simulink model "Intergration"  (R2018b)
settings: Solver=FixedStepDiscrete  StartTime=0.0  StopTime=inf  FixedStep=0.005  RelTol=1e-3
PostLoadFcn:
  | if any(exist('dsrtsu_mdlpostloadfcn', 'file') ~= 0), dsrtsu_mdlpostloadfcn('Execute', bdroot); end
values from neighbouring files (symbols this model uses):
  P_x165_On = 1.0    [CAN_Tx.sldd]
  P_x242_On = 1.0    [CAN_Tx.sldd]
  P_x246_On = 1.0    [CAN_Tx.sldd]
libraries: rtican x112, simulink x59
(part 13 of 31)

== system Intergration/Radar410_RX/x61_31 ==
  Bus Creator1 : BusCreator  Inputs=20
  FRS_Obj_17_Part1of2 : rtican/RTICAN Receive (RX)   Reserved1=[]  Reserved2=[]  Reserved3=[]  Reserved4=[]  SfcnMessage=[]  Msg_Struct=[]  BoardTypeNo=[]  BoardNo=[]  ChannelNo=[]  Parameters=[]  DialogFcn=[]  UnitName=[]  Revision=[]  UnitValues=[]  DSProperties=struct('RTI',struct('Version',uint32(5),'BlockType',struct('isSLSource',uint8(1),'isSLSink',uint8(1),'isHWSource',uint8(0),'isHWSink',uint8(0),'isSetup',uint8(0),'isInline',uint8(1),'isNonInline',uint8(0),'isInterrupt',uint8(0),'isChannelwise',uint8(0)),'IOBoardType','RTICAN','UnitType','MESSAGE','Identifier','RX','DialogType','MSVC','BlockSet','RTICAN','SlaveProcessor','CAN'))  RTIBlockInterface=struct('OutputPortsWidth',int32([1 1 1 1 1 1 1 1 1 1 1 1 1 1 1]),'OutputPortsActive',ones(1,15),'OutputPortsName',{{'FRS_P1_17_Msg_CheckSum','FRS_P1_17_Msg_AliveCounter','FRS_P1_17_Obj_ExstProb','FRS_P1_17_Obj_XVelRel_Stdev','FRS_P1_17_Obj_XAccRel','FRS_P1_17_Obj_ObstacleProb','FRS_P1_17_Obj_MotionPattern','FRS_P1_17_Obj_YPos_Stdev','FRS_P1_17_Obj_ValidFlag','FRS_P1_17_Obj_XPos_Stdev','FRS_P1_17_Obj_UpdateFlag','FRS_P1_17_Obj_ID',['RX status'],['RX time'],['RX delta time']}},'OutputPortsDataType',{{'SS_DOUBLE','SS_DOUBLE','SS_DOUBLE','SS_DOUBLE','SS_DOUBLE','SS_DOUBLE','SS_DOUBLE','SS_DOUBLE','SS_DOUBLE','SS_DOUBLE','SS_DOUBLE','SS_DOUBLE','SS_DOUBLE','SS_DOUBLE','SS_DOUBLE'}},'OutputPortsLabel',{{'FRS_P1_17_Msg_CheckSum','FRS_P1_17_Msg_AliveCounter','FRS_P1_17_Obj_ExstProb','FRS_P1_17_Obj_XVelRel_Stdev','FRS_P1_17_Obj_XAccRel','FRS_P1_17_Obj_ObstacleProb','FRS_P1_17_Obj_MotionPattern','FRS_P1_17_Obj_YPos_Stdev','FRS_P1_17_Obj_ValidFlag','FRS_P1_17_Obj_XPos_Stdev','FRS_P1_17_Obj_UpdateFlag','FRS_P1_17_Obj_ID','','',''}},'OutputPortsLabelMode','ON','InputPortsWidth',int32(0),'InputPortsActive',0,'DialogFcn','rtican_message_interface_gui','BlockDisplay',{{'','center'}},'IconTransparency','on','ParameterTunableNames',{{}},'InitLevel',3,'BlockName',struct('Token',{{'FRS_Obj_17_Part1of2'}}),'SampleTime',{{-1}},'TriggerPort',{{'none'}},'EnablePort',{{'none'}})  RTIBlockParameters=struct('BoardTypeNo',{{1,'OFF',[]}},'BoardNo',{{2,'ON',[1 16]}},'ChannelNo',{{2,'ON',[1 2]}},'Parameters',{{struct('DataFileSupport',struct('DataFileSelectedMaster',1,'DataFileSelectedLocal',1,'DataFileName','d:\00_work\00_zop\00_zop_demo_sim\asr410od_privatecan\privatecan\ars410od_privatecan.dbc|','DataFileDate',{{{['04-12月-2019 16:27:24']}}},'SelectedFile','asr410od_privatecan\privatecan\ars410od_privatecan.dbc'),'Options',struct('StatusSelected',1,'TimeSelected',1,'DeltaTimeSelected',1,'BytePortSelected',0,'MessageLengthSelected',0,'TriggerPort',struct('Selected',0,'TriggerType',0),'UserCoding',struct('Selected',0,'InterfaceFile','UserDecodingFile','FcnName','UserDecodeFcn','InportSelected',0,'InportWidth',1,'OutportSelected',0,'OutportWidth',1),'EnablePortSelected',0,'SignalOnPortnameSelected',1,'UseRXService',0),'Message',struct('MsgOnBlocknameSelected',1,'MsgName','FRS_Obj_17_Part1of2','MsgIdFormat',0,'MsgId',97,'MsgLength',8,'NumSignals',12,'SampleTime',-1,'Signal',struct('SgnName',{'FRS_P1_17_Msg_CheckSum','FRS_P1_17_Msg_AliveCounter','FRS_P1_17_Obj_ExstProb','FRS_P1_17_Obj_XVelRel_Stdev','FRS_P1_17_Obj_XAccRel','FRS_P1_17_Obj_ObstacleProb','FRS_P1_17_Obj_MotionPattern','FRS_P1_17_Obj_YPos_Stdev','FRS_P1_17_Obj_ValidFlag','FRS_P1_17_Obj_XPos_Stdev','FRS_P1_17_Obj_UpdateFlag','FRS_P1_17_Obj_ID'},'SgnStartBit',{0,8,12,18,25,32,37,40,47,48,55,56},'SgnLength',{8,4,6,7,7,5,3,7,1,7,1,8},'SgnType',{0,0,0,0,0,0,0,0,0,0,0,0},'ModeValue',{-1,-1,-1,-1,-1,-1,-1,-1,-1,-1,-1,-1},'DataType',{0,0,0,0,0,0,0,0,0,0,0,0},'ByteLayout',{2,2,2,2,2,2,2,2,2,2,2,2},'Factor',{1,1,1.5873,0.05,0.15,3.2258,1,0.1,1,0.1,1,1},'Offset',{0,0,0,0,-9.6,0,0,0,0,0,0,0},'SgnComment',{{['Check sum shall be generated out of each message content. check sum generation logic is TBC.']},{['Alive counter shall be incremented every radar sensor measurement cycle.']},{['Estimated existence probability of the object.']},{['Estimated 3-sigma standard deviation value of the relative longitudinal velocity of the object.']},{['Relative longitudinal acceleration of the object']},{['Estimated probability of the object being an obstacle.']},{['Motion type of object.' char(10) '0x00: Unknown' char(10) '0x01: Stationary' char(10) '0x02: Stopped' char(10) '0x03: Moving' char(10) '0x04: Crossing' char(10) '0x05-07: reserved']},{['Estimated 3-sigma standard deviation value of lateral position of the object.']},{['Validity indication flag. when this value shows invalid, all the signals in the corresponding CAN messages except FRS_Msg_AliveCounter and FRS_Msg_CheckSum shall take default values.' char(10) '0x0: Object invalid' char(10) '0x1: Object valid']},{['Estimated 3-sigma standard deviation value of longitudinal position of the object.']},{['Flag to indicate newly created object in CAN bus.' char(10) 'Object history flag' char(10) '0x0: new object in the cycle;' char(10) '0x1: object existed in previous cycle']},{['ID is defined as a unique identification number over the lifetime of the object.' char(10) '0xFF: Invalid' char(10) '0x00 - 0xFE: Valid']}},'SgnUnit',{'n/a','n/a','%','m/s','m/s2','%','n/a','m','n/a','m','n/a','n/a'},'Min',{0,0,0,0,-9.6,0,0,0,0,0,0,0},'Max',{255,15,99.9999,6.35,9.45,99.9998,7,12.7,1,12.7,1,255},'SLDataType',{'SS_DOUBLE','SS_DOUBLE','SS_DOUBLE','SS_DOUBLE','SS_DOUBLE','SS_DOUBLE','SS_DOUBLE','SS_DOUBLE','SS_DOUBLE','SS_DOUBLE','SS_DOUBLE','SS_DOUBLE'}),'MsgIdNumFormat',0,'MsgComment',{{''}}),'Version',1.2,'general',struct('isFromLib',0)),'OFF',[]}},'GroupId',{{struct('Group',{{'RTICAN'}},'No',2,'Behavior',{{'NAMECHANGE'}},'BlockType',{{'SINK'}},'NameChangeFlag',0),'OFF',[]}},'SFcnRTICANMessage',{{struct('MsgType','RX','SFcnPortType','Scalar','MsgName','FRS_Obj_17_Part1of2','MsgIdFormat','STD','MsgId',97,'MsgLength',8,'NumSignals',12,'SampleTime',-1,'Signal',struct('SgnName',{'FRS_P1_17_Msg_CheckSum','FRS_P1_17_Msg_AliveCounter','FRS_P1_17_Obj_ExstProb','FRS_P1_17_Obj_XVelRel_Stdev','FRS_P1_17_Obj_XAccRel','FRS_P1_17_Obj_ObstacleProb','FRS_P1_17_Obj_MotionPattern','FRS_P1_17_Obj_YPos_Stdev','FRS_P1_17_Obj_ValidFlag','FRS_P1_17_Obj_XPos_Stdev','FRS_P1_17_Obj_UpdateFlag','FRS_P1_17_Obj_ID'},'SgnStartBit',{0,8,12,18,25,32,37,40,47,48,55,56},'SgnLength',{8,4,6,7,7,5,3,7,1,7,1,8},'SgnType',{'standard','standard','standard','standard','standard','standard','standard','standard','standard','standard','standard','standard'},'ModeValue',{-1,-1,-1,-1,-1,-1,-1,-1,-1,-1,-1,-1},'DataType',{['unsigned int'],['unsigned int'],['unsigned int'],['unsigned int'],['unsigned int'],['unsigned int'],['unsigned int'],['unsigned int'],['unsigned int'],['unsigned int'],['unsigned int'],['unsigned int']},'ByteLayout',{['motorola back.'],['motorola back.'],['motorola back.'],['motorola back.'],['motorola back.'],['motorola back.'],['motorola back.'],['motorola back.'],['motorola back.'],['motorola back.'],['motorola back.'],['motorola back.']},'Factor',{1,1,1.5873,0.05,0.15,3.2258,1,0.1,1,0.1,1,1},'Offset',{0,0,0,0,-9.6,0,0,0,0,0,0,0},'SLDataType',{'SS_DOUBLE','SS_DOUBLE','SS_DOUBLE','SS_DOUBLE','SS_DOUBLE','SS_DOUBLE','SS_DOUBLE','SS_DOUBLE','SS_DOUBLE','SS_DOUBLE','SS_DOUBLE','SS_DOUBLE'}),'StatusSelected','yes','TimeSelected','yes','DeltaTimeSelected','yes','BytePortSelected','no','MessageLengthSelected','no','TriggerPort',struct('Selected','no','TriggerType',0),'UserCoding',struct('Selected','no','InterfaceFile','UserDecodingFile','FcnName','UserDecodeFcn','InportSelected','no','InportWidth',1,'OutportSelected','no','OutportWidth',1),'EnablePortSelected','no','UseRXService','no','BoardType','DS1','BoardNo',2,'ControllerNo',1),'OFF',[]}},'TLCFileName',{{'rtican_rx_message','OFF',[]}})  RTISFcnParameters=struct('SFcnRTICANMessage','struct','TLCFileName','char')  RTIBlockParaDefault=struct('BoardTypeNo',4302,'BoardNo',1,'ChannelNo',1,'Parameters',struct('DataFileSupport',struct('DataFileSelectedMaster',0,'DataFileSelectedLocal',0,'DataFileName','','DataFileDate','','SelectedFile',['<no file selected>']),'Options',struct('StatusSelected',1,'TimeSelected',1,'DeltaTimeSelected',1,'BytePortSelected',0,'MessageLengthSelected',0,'TriggerPort',struct('Selected',0,'TriggerType','rising'),'UserCoding',struct('Selected',0,'InterfaceFile','UserDecodingFile','FcnName','UserDecodeFcn','InportSelected',0,'InportWidth',1,'OutportSelected',0,'OutportWidth',1),'EnablePortSelected',0,'SignalOnPortnameSelected',1,'UseRXService',0),'Message',struct('MsgOnBlocknameSelected',0,'MsgName',['RX Message'],'MsgIdFormat',0,'MsgId',100,'MsgLength',8,'NumSignals',1,'SampleTime',-1,'Signal',struct('SgnName',['RX signal'],'SgnStartBit',0,'SgnLength',8,'SgnType',0,'ModeValue',-1,'DataType',0,'SLDataType','SS_DOUBLE','ByteLayout',0,'Factor',1,'Offset',0,'Min',0,'Max',255,'SgnComment',{{}},'SgnUnit',''),'MsgIdNumFormat',0,'MsgComment',{{''}}),'Version',1.2,'general',struct('isFromLib',1)),'GroupId',struct('Group',{{'RTICAN'}},'No',1,'Behavior',{{'NAMECHANGE'}},'BlockType',{{'SINK'}},'NameChangeFlag',0),'SFcnRTICANMessage',struct('MsgType','RX','MsgName',['RX Message'],'MsgIdFormat','STD','MsgId',100,'MsgLength',8,'NumSignals',1,'SampleTime',-1,'Signal',struct('SgnName',['RX signal'],'SgnStartBit',0,'SgnLength',8,'SgnType','standard','ModeValue',-1,'DataType',['unsigned int'],'ByteLayout',['little endian'],'SLDataType','SS_DOUBLE','Factor',1,'Offset',0),'StatusSelected','yes','TimeSelected','yes','DeltaTimeSelected','yes','BytePortSelected','no','MessageLengthSelected','no','EnablePortSelected','no','UserCoding',struct('Selected','no','InterfaceFile','UserDecodingFile','FcnName','UserDecodeFcn','InportSelected','no','InportWidth',1,'OutportSelected','no','OutportWidth',1),'TriggerPort',struct('Selected','no','TriggerType','rising'),'UseRXService','no','BoardType','DS4302','BoardNo',1,'ControllerNo',1,'SFcnPortType','Scalar'),'TLCFileName','rtican_rx_message')
      settings: AttributesFormatString=Group Id: RTICAN2\n  SourceProductName=dSPACE RTI CAN Blockset
  FRS_Obj_17_Part2of2 : rtican/RTICAN Receive (RX)   Reserved1=[]  Reserved2=[]  Reserved3=[]  Reserved4=[]  SfcnMessage=[]  Msg_Struct=[]  BoardTypeNo=[]  BoardNo=[]  ChannelNo=[]  Parameters=[]  DialogFcn=[]  UnitName=[]  Revision=[]  UnitValues=[]  DSProperties=struct('RTI',struct('Version',uint32(5),'BlockType',struct('isSLSource',uint8(1),'isSLSink',uint8(1),'isHWSource',uint8(0),'isHWSink',uint8(0),'isSetup',uint8(0),'isInline',uint8(1),'isNonInline',uint8(0),'isInterrupt',uint8(0),'isChannelwise',uint8(0)),'IOBoardType','RTICAN','UnitType','MESSAGE','Identifier','RX','DialogType','MSVC','BlockSet','RTICAN','SlaveProcessor','CAN'))  RTIBlockInterface=struct('OutputPortsWidth',int32([1 1 1 1 1 1 1 1 1 1 1]),'OutputPortsActive',ones(1,11),'OutputPortsName',{{'FRS_P2_17_Msg_CheckSum','FRS_P2_17_Msg_AliveCounter','FRS_P2_17_Obj_MeasFlag','FRS_P2_17_Obj_YVelRel','FRS_P2_17_Obj_Type','FRS_P2_17_Obj_XPos','FRS_P2_17_Obj_YPos','FRS_P2_17_Obj_XVelRel',['RX status'],['RX time'],['RX delta time']}},'OutputPortsDataType',{{'SS_DOUBLE','SS_DOUBLE','SS_DOUBLE','SS_DOUBLE','SS_DOUBLE','SS_DOUBLE','SS_DOUBLE','SS_DOUBLE','SS_DOUBLE','SS_DOUBLE','SS_DOUBLE'}},'OutputPortsLabel',{{'FRS_P2_17_Msg_CheckSum','FRS_P2_17_Msg_AliveCounter','FRS_P2_17_Obj_MeasFlag','FRS_P2_17_Obj_YVelRel','FRS_P2_17_Obj_Type','FRS_P2_17_Obj_XPos','FRS_P2_17_Obj_YPos','FRS_P2_17_Obj_XVelRel','','',''}},'OutputPortsLabelMode','ON','InputPortsWidth',int32(0),'InputPortsActive',0,'DialogFcn','rtican_message_interface_gui','BlockDisplay',{{'','center'}},'IconTransparency','on','ParameterTunableNames',{{}},'InitLevel',3,'BlockName',struct('Token',{{'FRS_Obj_17_Part2of2'}}),'SampleTime',{{-1}},'TriggerPort',{{'none'}},'EnablePort',{{'none'}})  RTIBlockParameters=struct('BoardTypeNo',{{1,'OFF',[]}},'BoardNo',{{2,'ON',[1 16]}},'ChannelNo',{{2,'ON',[1 2]}},'Parameters',{{struct('DataFileSupport',struct('DataFileSelectedMaster',1,'DataFileSelectedLocal',1,'DataFileName','d:\00_work\00_zop\00_zop_demo_sim\asr410od_privatecan\privatecan\ars410od_privatecan.dbc|','DataFileDate',{{{['04-12月-2019 16:27:24']}}},'SelectedFile','asr410od_privatecan\privatecan\ars410od_privatecan.dbc'),'Options',struct('StatusSelected',1,'TimeSelected',1,'DeltaTimeSelected',1,'BytePortSelected',0,'MessageLengthSelected',0,'TriggerPort',struct('Selected',0,'TriggerType',0),'UserCoding',struct('Selected',0,'InterfaceFile','UserDecodingFile','FcnName','UserDecodeFcn','InportSelected',0,'InportWidth',1,'OutportSelected',0,'OutportWidth',1),'EnablePortSelected',0,'SignalOnPortnameSelected',1,'UseRXService',0),'Message',struct('MsgOnBlocknameSelected',1,'MsgName','FRS_Obj_17_Part2of2','MsgIdFormat',0,'MsgId',49,'MsgLength',8,'NumSignals',8,'SampleTime',-1,'Signal',struct('SgnName',{'FRS_P2_17_Msg_CheckSum','FRS_P2_17_Msg_AliveCounter','FRS_P2_17_Obj_MeasFlag','FRS_P2_17_Obj_YVelRel','FRS_P2_17_Obj_Type','FRS_P2_17_Obj_XPos','FRS_P2_17_Obj_YPos','FRS_P2_17_Obj_XVelRel'},'SgnStartBit',{0,8,12,13,24,26,40,53},'SgnLength',{8,4,1,11,2,14,13,11},'SgnType',{0,0,0,0,0,0,0,0},'ModeValue',{-1,-1,-1,-1,-1,-1,-1,-1},'DataType',{0,0,0,0,0,0,0,0},'ByteLayout',{2,2,2,2,2,2,2,2},'Factor',{1,1,1,0.1,1,2^-6,2^-6,0.1},'Offset',{0,0,0,-102.4,0,0,-64,-102.4},'SgnComment',{{['Check sum shall be generated out of each message content. check sum generation logic is TBC.']},{['Alive counter shall be incremented every radar sensor measurement cycle.']},{['This signal indicates whether the latest sensor measurement observed the object or extrapolated.' char(10) '0x0: object measured in this cycle' char(10) '0x1: object extrapolated in this cycle']},{['Relative lateral velocity of the object']},{['To indicate the estimated type of Object' char(10) '0x00: Unknown' char(10) '0x01: 4 wheeler' char(10) '0x02: 2 wheeler' char(10) '0x03: Pedestrian']},{['Position of target object in longitudinal direction' char(10) 'center of vehicle rear axle shaft is reference point.']},{['Position of target object in lateral direction' char(10) 'center of vehicle rear axle shaft is reference point.']},{['Relative longitudinal velocity of the object.']}},'SgnUnit',{'n/a','n/a','n/a','m/s','n/a','m','m','m/s'},'Min',{0,0,0,-102.4,0,0,-64,-102.4},'Max',{255,15,1,102.3,3,255.984375,63.984375,102.3},'SLDataType',{'SS_DOUBLE','SS_DOUBLE','SS_DOUBLE','SS_DOUBLE','SS_DOUBLE','SS_DOUBLE','SS_DOUBLE','SS_DOUBLE'}),'MsgIdNumFormat',0,'MsgComment',{{''}}),'Version',1.2,'general',struct('isFromLib',0)),'OFF',[]}},'GroupId',{{struct('Group',{{'RTICAN'}},'No',2,'Behavior',{{'NAMECHANGE'}},'BlockType',{{'SINK'}},'NameChangeFlag',0),'OFF',[]}},'SFcnRTICANMessage',{{struct('MsgType','RX','SFcnPortType','Scalar','MsgName','FRS_Obj_17_Part2of2','MsgIdFormat','STD','MsgId',49,'MsgLength',8,'NumSignals',8,'SampleTime',-1,'Signal',struct('SgnName',{'FRS_P2_17_Msg_CheckSum','FRS_P2_17_Msg_AliveCounter','FRS_P2_17_Obj_MeasFlag','FRS_P2_17_Obj_YVelRel','FRS_P2_17_Obj_Type','FRS_P2_17_Obj_XPos','FRS_P2_17_Obj_YPos','FRS_P2_17_Obj_XVelRel'},'SgnStartBit',{0,8,12,13,24,26,40,53},'SgnLength',{8,4,1,11,2,14,13,11},'SgnType',{'standard','standard','standard','standard','standard','standard','standard','standard'},'ModeValue',{-1,-1,-1,-1,-1,-1,-1,-1},'DataType',{['unsigned int'],['unsigned int'],['unsigned int'],['unsigned int'],['unsigned int'],['unsigned int'],['unsigned int'],['unsigned int']},'ByteLayout',{['motorola back.'],['motorola back.'],['motorola back.'],['motorola back.'],['motorola back.'],['motorola back.'],['motorola back.'],['motorola back.']},'Factor',{1,1,1,0.1,1,2^-6,2^-6,0.1},'Offset',{0,0,0,-102.4,0,0,-64,-102.4},'SLDataType',{'SS_DOUBLE','SS_DOUBLE','SS_DOUBLE','SS_DOUBLE','SS_DOUBLE','SS_DOUBLE','SS_DOUBLE','SS_DOUBLE'}),'StatusSelected','yes','TimeSelected','yes','DeltaTimeSelected','yes','BytePortSelected','no','MessageLengthSelected','no','TriggerPort',struct('Selected','no','TriggerType',0),'UserCoding',struct('Selected','no','InterfaceFile','UserDecodingFile','FcnName','UserDecodeFcn','InportSelected','no','InportWidth',1,'OutportSelected','no','OutportWidth',1),'EnablePortSelected','no','UseRXService','no','BoardType','DS1','BoardNo',2,'ControllerNo',1),'OFF',[]}},'TLCFileName',{{'rtican_rx_message','OFF',[]}})  RTISFcnParameters=struct('SFcnRTICANMessage','struct','TLCFileName','char')  RTIBlockParaDefault=struct('BoardTypeNo',4302,'BoardNo',1,'ChannelNo',1,'Parameters',struct('DataFileSupport',struct('DataFileSelectedMaster',0,'DataFileSelectedLocal',0,'DataFileName','','DataFileDate','','SelectedFile',['<no file selected>']),'Options',struct('StatusSelected',1,'TimeSelected',1,'DeltaTimeSelected',1,'BytePortSelected',0,'MessageLengthSelected',0,'TriggerPort',struct('Selected',0,'TriggerType','rising'),'UserCoding',struct('Selected',0,'InterfaceFile','UserDecodingFile','FcnName','UserDecodeFcn','InportSelected',0,'InportWidth',1,'OutportSelected',0,'OutportWidth',1),'EnablePortSelected',0,'SignalOnPortnameSelected',1,'UseRXService',0),'Message',struct('MsgOnBlocknameSelected',0,'MsgName',['RX Message'],'MsgIdFormat',0,'MsgId',100,'MsgLength',8,'NumSignals',1,'SampleTime',-1,'Signal',struct('SgnName',['RX signal'],'SgnStartBit',0,'SgnLength',8,'SgnType',0,'ModeValue',-1,'DataType',0,'SLDataType','SS_DOUBLE','ByteLayout',0,'Factor',1,'Offset',0,'Min',0,'Max',255,'SgnComment',{{}},'SgnUnit',''),'MsgIdNumFormat',0,'MsgComment',{{''}}),'Version',1.2,'general',struct('isFromLib',1)),'GroupId',struct('Group',{{'RTICAN'}},'No',1,'Behavior',{{'NAMECHANGE'}},'BlockType',{{'SINK'}},'NameChangeFlag',0),'SFcnRTICANMessage',struct('MsgType','RX','MsgName',['RX Message'],'MsgIdFormat','STD','MsgId',100,'MsgLength',8,'NumSignals',1,'SampleTime',-1,'Signal',struct('SgnName',['RX signal'],'SgnStartBit',0,'SgnLength',8,'SgnType','standard','ModeValue',-1,'DataType',['unsigned int'],'ByteLayout',['little endian'],'SLDataType','SS_DOUBLE','Factor',1,'Offset',0),'StatusSelected','yes','TimeSelected','yes','DeltaTimeSelected','yes','BytePortSelected','no','MessageLengthSelected','no','EnablePortSelected','no','UserCoding',struct('Selected','no','InterfaceFile','UserDecodingFile','FcnName','UserDecodeFcn','InportSelected','no','InportWidth',1,'OutportSelected','no','OutportWidth',1),'TriggerPort',struct('Selected','no','TriggerType','rising'),'UseRXService','no','BoardType','DS4302','BoardNo',1,'ControllerNo',1,'SFcnPortType','Scalar'),'TLCFileName','rtican_rx_message')
      settings: AttributesFormatString=Group Id: RTICAN2\n  SourceProductName=dSPACE RTI CAN Blockset
  Terminator{,1..5} (6 alike) : Terminator
  Out1 : Outport
  wires:
  Bus Creator1/1 -> Out1/1
  FRS_Obj_17_Part2of2/11 -> Terminator5/1
  FRS_Obj_17_Part2of2/9 -> Terminator3/1
  FRS_Obj_17_Part2of2/10 -> Terminator4/1
  FRS_Obj_17_Part1of2/13 -> Terminator/1
  FRS_Obj_17_Part1of2/14 -> Terminator1/1
  FRS_Obj_17_Part1of2/15 -> Terminator2/1
  FRS_Obj_17_Part1of2/1 -> Bus Creator1/1  "FRS_P1_17_Msg_CheckSum"
  FRS_Obj_17_Part1of2/2 -> Bus Creator1/2  "FRS_P1_17_Msg_AliveCounter"
  FRS_Obj_17_Part1of2/3 -> Bus Creator1/3  "FRS_P1_17_Obj_ExstProb"
  FRS_Obj_17_Part1of2/4 -> Bus Creator1/4  "FRS_P1_17_Obj_XVelRel_Stdev"
  FRS_Obj_17_Part1of2/5 -> Bus Creator1/5  "FRS_P1_17_Obj_XAccRel"
  FRS_Obj_17_Part1of2/6 -> Bus Creator1/6  "FRS_P1_17_Obj_ObstacleProb"
  FRS_Obj_17_Part1of2/7 -> Bus Creator1/7  "FRS_P1_17_Obj_MotionPattern"
  FRS_Obj_17_Part1of2/8 -> Bus Creator1/8  "FRS_P1_17_Obj_YPos_Stdev"
  FRS_Obj_17_Part1of2/9 -> Bus Creator1/9  "FRS_P1_17_Obj_ValidFlag"
  FRS_Obj_17_Part1of2/10 -> Bus Creator1/10  "FRS_P1_17_Obj_XPos_Stdev"
  FRS_Obj_17_Part1of2/11 -> Bus Creator1/11  "FRS_P1_17_Obj_UpdateFlag"
  FRS_Obj_17_Part1of2/12 -> Bus Creator1/12  "FRS_P1_17_Obj_ID"
  FRS_Obj_17_Part2of2/8 -> Bus Creator1/20  "FRS_P2_17_Obj_XVelRel"
  FRS_Obj_17_Part2of2/7 -> Bus Creator1/19  "FRS_P2_17_Obj_YPos"
  FRS_Obj_17_Part2of2/6 -> Bus Creator1/18  "FRS_P2_17_Obj_XPos"
  FRS_Obj_17_Part2of2/5 -> Bus Creator1/17  "FRS_P2_17_Obj_Type"
  FRS_Obj_17_Part2of2/4 -> Bus Creator1/16  "FRS_P2_17_Obj_YVelRel"
  FRS_Obj_17_Part2of2/3 -> Bus Creator1/15  "FRS_P2_17_Obj_MeasFlag"
  FRS_Obj_17_Part2of2/2 -> Bus Creator1/14  "FRS_P2_17_Msg_AliveCounter"
  FRS_Obj_17_Part2of2/1 -> Bus Creator1/13  "FRS_P2_17_Msg_CheckSum"

== system Intergration/Radar410_RX/x62_32 ==
  Bus Creator1 : BusCreator  Inputs=20
  FRS_Obj_18_Part1of2 : rtican/RTICAN Receive (RX)   Reserved1=[]  Reserved2=[]  Reserved3=[]  Reserved4=[]  SfcnMessage=[]  Msg_Struct=[]  BoardTypeNo=[]  BoardNo=[]  ChannelNo=[]  Parameters=[]  DialogFcn=[]  UnitName=[]  Revision=[]  UnitValues=[]  DSProperties=struct('RTI',struct('Version',uint32(5),'BlockType',struct('isSLSource',uint8(1),'isSLSink',uint8(1),'isHWSource',uint8(0),'isHWSink',uint8(0),'isSetup',uint8(0),'isInline',uint8(1),'isNonInline',uint8(0),'isInterrupt',uint8(0),'isChannelwise',uint8(0)),'IOBoardType','RTICAN','UnitType','MESSAGE','Identifier','RX','DialogType','MSVC','BlockSet','RTICAN','SlaveProcessor','CAN'))  RTIBlockInterface=struct('OutputPortsWidth',int32([1 1 1 1 1 1 1 1 1 1 1 1 1 1 1]),'OutputPortsActive',ones(1,15),'OutputPortsName',{{'FRS_P1_18_Msg_CheckSum','FRS_P1_18_Msg_AliveCounter','FRS_P1_18_Obj_ExstProb','FRS_P1_18_Obj_XVelRel_Stdev','FRS_P1_18_Obj_XAccRel','FRS_P1_18_Obj_ObstacleProb','FRS_P1_18_Obj_MotionPattern','FRS_P1_18_Obj_YPos_Stdev','FRS_P1_18_Obj_ValidFlag','FRS_P1_18_Obj_XPos_Stdev','FRS_P1_18_Obj_UpdateFlag','FRS_P1_18_Obj_ID',['RX status'],['RX time'],['RX delta time']}},'OutputPortsDataType',{{'SS_DOUBLE','SS_DOUBLE','SS_DOUBLE','SS_DOUBLE','SS_DOUBLE','SS_DOUBLE','SS_DOUBLE','SS_DOUBLE','SS_DOUBLE','SS_DOUBLE','SS_DOUBLE','SS_DOUBLE','SS_DOUBLE','SS_DOUBLE','SS_DOUBLE'}},'OutputPortsLabel',{{'FRS_P1_18_Msg_CheckSum','FRS_P1_18_Msg_AliveCounter','FRS_P1_18_Obj_ExstProb','FRS_P1_18_Obj_XVelRel_Stdev','FRS_P1_18_Obj_XAccRel','FRS_P1_18_Obj_ObstacleProb','FRS_P1_18_Obj_MotionPattern','FRS_P1_18_Obj_YPos_Stdev','FRS_P1_18_Obj_ValidFlag','FRS_P1_18_Obj_XPos_Stdev','FRS_P1_18_Obj_UpdateFlag','FRS_P1_18_Obj_ID','','',''}},'OutputPortsLabelMode','ON','InputPortsWidth',int32(0),'InputPortsActive',0,'DialogFcn','rtican_message_interface_gui','BlockDisplay',{{'','center'}},'IconTransparency','on','ParameterTunableNames',{{}},'InitLevel',3,'BlockName',struct('Token',{{'FRS_Obj_18_Part1of2'}}),'SampleTime',{{-1}},'TriggerPort',{{'none'}},'EnablePort',{{'none'}})  RTIBlockParameters=struct('BoardTypeNo',{{1,'OFF',[]}},'BoardNo',{{2,'ON',[1 16]}},'ChannelNo',{{2,'ON',[1 2]}},'Parameters',{{struct('DataFileSupport',struct('DataFileSelectedMaster',1,'DataFileSelectedLocal',1,'DataFileName','d:\00_work\00_zop\00_zop_demo_sim\asr410od_privatecan\privatecan\ars410od_privatecan.dbc|','DataFileDate',{{{['04-12月-2019 16:27:24']}}},'SelectedFile','asr410od_privatecan\privatecan\ars410od_privatecan.dbc'),'Options',struct('StatusSelected',1,'TimeSelected',1,'DeltaTimeSelected',1,'BytePortSelected',0,'MessageLengthSelected',0,'TriggerPort',struct('Selected',0,'TriggerType',0),'UserCoding',struct('Selected',0,'InterfaceFile','UserDecodingFile','FcnName','UserDecodeFcn','InportSelected',0,'InportWidth',1,'OutportSelected',0,'OutportWidth',1),'EnablePortSelected',0,'SignalOnPortnameSelected',1,'UseRXService',0),'Message',struct('MsgOnBlocknameSelected',1,'MsgName','FRS_Obj_18_Part1of2','MsgIdFormat',0,'MsgId',98,'MsgLength',8,'NumSignals',12,'SampleTime',-1,'Signal',struct('SgnName',{'FRS_P1_18_Msg_CheckSum','FRS_P1_18_Msg_AliveCounter','FRS_P1_18_Obj_ExstProb','FRS_P1_18_Obj_XVelRel_Stdev','FRS_P1_18_Obj_XAccRel','FRS_P1_18_Obj_ObstacleProb','FRS_P1_18_Obj_MotionPattern','FRS_P1_18_Obj_YPos_Stdev','FRS_P1_18_Obj_ValidFlag','FRS_P1_18_Obj_XPos_Stdev','FRS_P1_18_Obj_UpdateFlag','FRS_P1_18_Obj_ID'},'SgnStartBit',{0,8,12,18,25,32,37,40,47,48,55,56},'SgnLength',{8,4,6,7,7,5,3,7,1,7,1,8},'SgnType',{0,0,0,0,0,0,0,0,0,0,0,0},'ModeValue',{-1,-1,-1,-1,-1,-1,-1,-1,-1,-1,-1,-1},'DataType',{0,0,0,0,0,0,0,0,0,0,0,0},'ByteLayout',{2,2,2,2,2,2,2,2,2,2,2,2},'Factor',{1,1,1.5873,0.05,0.15,3.2258,1,0.1,1,0.1,1,1},'Offset',{0,0,0,0,-9.6,0,0,0,0,0,0,0},'SgnComment',{{['Check sum shall be generated out of each message content. check sum generation logic is TBC.']},{['Alive counter shall be incremented every radar sensor measurement cycle.']},{['Estimated existence probability of the object.']},{['Estimated 3-sigma standard deviation value of the relative longitudinal velocity of the object.']},{['Relative longitudinal acceleration of the object']},{['Estimated probability of the object being an obstacle.']},{['Motion type of object.' char(10) '0x00: Unknown' char(10) '0x01: Stationary' char(10) '0x02: Stopped' char(10) '0x03: Moving' char(10) '0x04: Crossing' char(10) '0x05-07: reserved']},{['Estimated 3-sigma standard deviation value of lateral position of the object.']},{['Validity indication flag. when this value shows invalid, all the signals in the corresponding CAN messages except FRS_Msg_AliveCounter and FRS_Msg_CheckSum shall take default values.' char(10) '0x0: Object invalid' char(10) '0x1: Object valid']},{['Estimated 3-sigma standard deviation value of longitudinal position of the object.']},{['Flag to indicate newly created object in CAN bus.' char(10) 'Object history flag' char(10) '0x0: new object in the cycle;' char(10) '0x1: object existed in previous cycle']},{['ID is defined as a unique identification number over the lifetime of the object.' char(10) '0xFF: Invalid' char(10) '0x00 - 0xFE: Valid']}},'SgnUnit',{'n/a','n/a','%','m/s','m/s2','%','n/a','m','n/a','m','n/a','n/a'},'Min',{0,0,0,0,-9.6,0,0,0,0,0,0,0},'Max',{255,15,99.9999,6.35,9.45,99.9998,7,12.7,1,12.7,1,255},'SLDataType',{'SS_DOUBLE','SS_DOUBLE','SS_DOUBLE','SS_DOUBLE','SS_DOUBLE','SS_DOUBLE','SS_DOUBLE','SS_DOUBLE','SS_DOUBLE','SS_DOUBLE','SS_DOUBLE','SS_DOUBLE'}),'MsgIdNumFormat',0,'MsgComment',{{''}}),'Version',1.2,'general',struct('isFromLib',0)),'OFF',[]}},'GroupId',{{struct('Group',{{'RTICAN'}},'No',2,'Behavior',{{'NAMECHANGE'}},'BlockType',{{'SINK'}},'NameChangeFlag',0),'OFF',[]}},'SFcnRTICANMessage',{{struct('MsgType','RX','SFcnPortType','Scalar','MsgName','FRS_Obj_18_Part1of2','MsgIdFormat','STD','MsgId',98,'MsgLength',8,'NumSignals',12,'SampleTime',-1,'Signal',struct('SgnName',{'FRS_P1_18_Msg_CheckSum','FRS_P1_18_Msg_AliveCounter','FRS_P1_18_Obj_ExstProb','FRS_P1_18_Obj_XVelRel_Stdev','FRS_P1_18_Obj_XAccRel','FRS_P1_18_Obj_ObstacleProb','FRS_P1_18_Obj_MotionPattern','FRS_P1_18_Obj_YPos_Stdev','FRS_P1_18_Obj_ValidFlag','FRS_P1_18_Obj_XPos_Stdev','FRS_P1_18_Obj_UpdateFlag','FRS_P1_18_Obj_ID'},'SgnStartBit',{0,8,12,18,25,32,37,40,47,48,55,56},'SgnLength',{8,4,6,7,7,5,3,7,1,7,1,8},'SgnType',{'standard','standard','standard','standard','standard','standard','standard','standard','standard','standard','standard','standard'},'ModeValue',{-1,-1,-1,-1,-1,-1,-1,-1,-1,-1,-1,-1},'DataType',{['unsigned int'],['unsigned int'],['unsigned int'],['unsigned int'],['unsigned int'],['unsigned int'],['unsigned int'],['unsigned int'],['unsigned int'],['unsigned int'],['unsigned int'],['unsigned int']},'ByteLayout',{['motorola back.'],['motorola back.'],['motorola back.'],['motorola back.'],['motorola back.'],['motorola back.'],['motorola back.'],['motorola back.'],['motorola back.'],['motorola back.'],['motorola back.'],['motorola back.']},'Factor',{1,1,1.5873,0.05,0.15,3.2258,1,0.1,1,0.1,1,1},'Offset',{0,0,0,0,-9.6,0,0,0,0,0,0,0},'SLDataType',{'SS_DOUBLE','SS_DOUBLE','SS_DOUBLE','SS_DOUBLE','SS_DOUBLE','SS_DOUBLE','SS_DOUBLE','SS_DOUBLE','SS_DOUBLE','SS_DOUBLE','SS_DOUBLE','SS_DOUBLE'}),'StatusSelected','yes','TimeSelected','yes','DeltaTimeSelected','yes','BytePortSelected','no','MessageLengthSelected','no','TriggerPort',struct('Selected','no','TriggerType',0),'UserCoding',struct('Selected','no','InterfaceFile','UserDecodingFile','FcnName','UserDecodeFcn','InportSelected','no','InportWidth',1,'OutportSelected','no','OutportWidth',1),'EnablePortSelected','no','UseRXService','no','BoardType','DS1','BoardNo',2,'ControllerNo',1),'OFF',[]}},'TLCFileName',{{'rtican_rx_message','OFF',[]}})  RTISFcnParameters=struct('SFcnRTICANMessage','struct','TLCFileName','char')  RTIBlockParaDefault=struct('BoardTypeNo',4302,'BoardNo',1,'ChannelNo',1,'Parameters',struct('DataFileSupport',struct('DataFileSelectedMaster',0,'DataFileSelectedLocal',0,'DataFileName','','DataFileDate','','SelectedFile',['<no file selected>']),'Options',struct('StatusSelected',1,'TimeSelected',1,'DeltaTimeSelected',1,'BytePortSelected',0,'MessageLengthSelected',0,'TriggerPort',struct('Selected',0,'TriggerType','rising'),'UserCoding',struct('Selected',0,'InterfaceFile','UserDecodingFile','FcnName','UserDecodeFcn','InportSelected',0,'InportWidth',1,'OutportSelected',0,'OutportWidth',1),'EnablePortSelected',0,'SignalOnPortnameSelected',1,'UseRXService',0),'Message',struct('MsgOnBlocknameSelected',0,'MsgName',['RX Message'],'MsgIdFormat',0,'MsgId',100,'MsgLength',8,'NumSignals',1,'SampleTime',-1,'Signal',struct('SgnName',['RX signal'],'SgnStartBit',0,'SgnLength',8,'SgnType',0,'ModeValue',-1,'DataType',0,'SLDataType','SS_DOUBLE','ByteLayout',0,'Factor',1,'Offset',0,'Min',0,'Max',255,'SgnComment',{{}},'SgnUnit',''),'MsgIdNumFormat',0,'MsgComment',{{''}}),'Version',1.2,'general',struct('isFromLib',1)),'GroupId',struct('Group',{{'RTICAN'}},'No',1,'Behavior',{{'NAMECHANGE'}},'BlockType',{{'SINK'}},'NameChangeFlag',0),'SFcnRTICANMessage',struct('MsgType','RX','MsgName',['RX Message'],'MsgIdFormat','STD','MsgId',100,'MsgLength',8,'NumSignals',1,'SampleTime',-1,'Signal',struct('SgnName',['RX signal'],'SgnStartBit',0,'SgnLength',8,'SgnType','standard','ModeValue',-1,'DataType',['unsigned int'],'ByteLayout',['little endian'],'SLDataType','SS_DOUBLE','Factor',1,'Offset',0),'StatusSelected','yes','TimeSelected','yes','DeltaTimeSelected','yes','BytePortSelected','no','MessageLengthSelected','no','EnablePortSelected','no','UserCoding',struct('Selected','no','InterfaceFile','UserDecodingFile','FcnName','UserDecodeFcn','InportSelected','no','InportWidth',1,'OutportSelected','no','OutportWidth',1),'TriggerPort',struct('Selected','no','TriggerType','rising'),'UseRXService','no','BoardType','DS4302','BoardNo',1,'ControllerNo',1,'SFcnPortType','Scalar'),'TLCFileName','rtican_rx_message')
      settings: AttributesFormatString=Group Id: RTICAN2\n  SourceProductName=dSPACE RTI CAN Blockset
  FRS_Obj_18_Part2of2 : rtican/RTICAN Receive (RX)   Reserved1=[]  Reserved2=[]  Reserved3=[]  Reserved4=[]  SfcnMessage=[]  Msg_Struct=[]  BoardTypeNo=[]  BoardNo=[]  ChannelNo=[]  Parameters=[]  DialogFcn=[]  UnitName=[]  Revision=[]  UnitValues=[]  DSProperties=struct('RTI',struct('Version',uint32(5),'BlockType',struct('isSLSource',uint8(1),'isSLSink',uint8(1),'isHWSource',uint8(0),'isHWSink',uint8(0),'isSetup',uint8(0),'isInline',uint8(1),'isNonInline',uint8(0),'isInterrupt',uint8(0),'isChannelwise',uint8(0)),'IOBoardType','RTICAN','UnitType','MESSAGE','Identifier','RX','DialogType','MSVC','BlockSet','RTICAN','SlaveProcessor','CAN'))  RTIBlockInterface=struct('OutputPortsWidth',int32([1 1 1 1 1 1 1 1 1 1 1]),'OutputPortsActive',ones(1,11),'OutputPortsName',{{'FRS_P2_18_Msg_CheckSum','FRS_P2_18_Msg_AliveCounter','FRS_P2_18_Obj_MeasFlag','FRS_P2_18_Obj_YVelRel','FRS_P2_18_Obj_Type','FRS_P2_18_Obj_XPos','FRS_P2_18_Obj_YPos','FRS_P2_18_Obj_XVelRel',['RX status'],['RX time'],['RX delta time']}},'OutputPortsDataType',{{'SS_DOUBLE','SS_DOUBLE','SS_DOUBLE','SS_DOUBLE','SS_DOUBLE','SS_DOUBLE','SS_DOUBLE','SS_DOUBLE','SS_DOUBLE','SS_DOUBLE','SS_DOUBLE'}},'OutputPortsLabel',{{'FRS_P2_18_Msg_CheckSum','FRS_P2_18_Msg_AliveCounter','FRS_P2_18_Obj_MeasFlag','FRS_P2_18_Obj_YVelRel','FRS_P2_18_Obj_Type','FRS_P2_18_Obj_XPos','FRS_P2_18_Obj_YPos','FRS_P2_18_Obj_XVelRel','','',''}},'OutputPortsLabelMode','ON','InputPortsWidth',int32(0),'InputPortsActive',0,'DialogFcn','rtican_message_interface_gui','BlockDisplay',{{'','center'}},'IconTransparency','on','ParameterTunableNames',{{}},'InitLevel',3,'BlockName',struct('Token',{{'FRS_Obj_18_Part2of2'}}),'SampleTime',{{-1}},'TriggerPort',{{'none'}},'EnablePort',{{'none'}})  RTIBlockParameters=struct('BoardTypeNo',{{1,'OFF',[]}},'BoardNo',{{2,'ON',[1 16]}},'ChannelNo',{{2,'ON',[1 2]}},'Parameters',{{struct('DataFileSupport',struct('DataFileSelectedMaster',1,'DataFileSelectedLocal',1,'DataFileName','d:\00_work\00_zop\00_zop_demo_sim\asr410od_privatecan\privatecan\ars410od_privatecan.dbc|','DataFileDate',{{{['04-12月-2019 16:27:24']}}},'SelectedFile','asr410od_privatecan\privatecan\ars410od_privatecan.dbc'),'Options',struct('StatusSelected',1,'TimeSelected',1,'DeltaTimeSelected',1,'BytePortSelected',0,'MessageLengthSelected',0,'TriggerPort',struct('Selected',0,'TriggerType',0),'UserCoding',struct('Selected',0,'InterfaceFile','UserDecodingFile','FcnName','UserDecodeFcn','InportSelected',0,'InportWidth',1,'OutportSelected',0,'OutportWidth',1),'EnablePortSelected',0,'SignalOnPortnameSelected',1,'UseRXService',0),'Message',struct('MsgOnBlocknameSelected',1,'MsgName','FRS_Obj_18_Part2of2','MsgIdFormat',0,'MsgId',50,'MsgLength',8,'NumSignals',8,'SampleTime',-1,'Signal',struct('SgnName',{'FRS_P2_18_Msg_CheckSum','FRS_P2_18_Msg_AliveCounter','FRS_P2_18_Obj_MeasFlag','FRS_P2_18_Obj_YVelRel','FRS_P2_18_Obj_Type','FRS_P2_18_Obj_XPos','FRS_P2_18_Obj_YPos','FRS_P2_18_Obj_XVelRel'},'SgnStartBit',{0,8,12,13,24,26,40,53},'SgnLength',{8,4,1,11,2,14,13,11},'SgnType',{0,0,0,0,0,0,0,0},'ModeValue',{-1,-1,-1,-1,-1,-1,-1,-1},'DataType',{0,0,0,0,0,0,0,0},'ByteLayout',{2,2,2,2,2,2,2,2},'Factor',{1,1,1,0.1,1,2^-6,2^-6,0.1},'Offset',{0,0,0,-102.4,0,0,-64,-102.4},'SgnComment',{{['Check sum shall be generated out of each message content. check sum generation logic is TBC.']},{['Alive counter shall be incremented every radar sensor measurement cycle.']},{['This signal indicates whether the latest sensor measurement observed the object or extrapolated.' char(10) '0x0: object measured in this cycle' char(10) '0x1: object extrapolated in this cycle']},{['Relative lateral velocity of the object']},{['To indicate the estimated type of Object' char(10) '0x00: Unknown' char(10) '0x01: 4 wheeler' char(10) '0x02: 2 wheeler' char(10) '0x03: Pedestrian']},{['Position of target object in longitudinal direction' char(10) 'center of vehicle rear axle shaft is reference point.']},{['Position of target object in lateral direction' char(10) 'center of vehicle rear axle shaft is reference point.']},{['Relative longitudinal velocity of the object.']}},'SgnUnit',{'n/a','n/a','n/a','m/s','n/a','m','m','m/s'},'Min',{0,0,0,-102.4,0,0,-64,-102.4},'Max',{255,15,1,102.3,3,255.984375,63.984375,102.3},'SLDataType',{'SS_DOUBLE','SS_DOUBLE','SS_DOUBLE','SS_DOUBLE','SS_DOUBLE','SS_DOUBLE','SS_DOUBLE','SS_DOUBLE'}),'MsgIdNumFormat',0,'MsgComment',{{''}}),'Version',1.2,'general',struct('isFromLib',0)),'OFF',[]}},'GroupId',{{struct('Group',{{'RTICAN'}},'No',2,'Behavior',{{'NAMECHANGE'}},'BlockType',{{'SINK'}},'NameChangeFlag',0),'OFF',[]}},'SFcnRTICANMessage',{{struct('MsgType','RX','SFcnPortType','Scalar','MsgName','FRS_Obj_18_Part2of2','MsgIdFormat','STD','MsgId',50,'MsgLength',8,'NumSignals',8,'SampleTime',-1,'Signal',struct('SgnName',{'FRS_P2_18_Msg_CheckSum','FRS_P2_18_Msg_AliveCounter','FRS_P2_18_Obj_MeasFlag','FRS_P2_18_Obj_YVelRel','FRS_P2_18_Obj_Type','FRS_P2_18_Obj_XPos','FRS_P2_18_Obj_YPos','FRS_P2_18_Obj_XVelRel'},'SgnStartBit',{0,8,12,13,24,26,40,53},'SgnLength',{8,4,1,11,2,14,13,11},'SgnType',{'standard','standard','standard','standard','standard','standard','standard','standard'},'ModeValue',{-1,-1,-1,-1,-1,-1,-1,-1},'DataType',{['unsigned int'],['unsigned int'],['unsigned int'],['unsigned int'],['unsigned int'],['unsigned int'],['unsigned int'],['unsigned int']},'ByteLayout',{['motorola back.'],['motorola back.'],['motorola back.'],['motorola back.'],['motorola back.'],['motorola back.'],['motorola back.'],['motorola back.']},'Factor',{1,1,1,0.1,1,2^-6,2^-6,0.1},'Offset',{0,0,0,-102.4,0,0,-64,-102.4},'SLDataType',{'SS_DOUBLE','SS_DOUBLE','SS_DOUBLE','SS_DOUBLE','SS_DOUBLE','SS_DOUBLE','SS_DOUBLE','SS_DOUBLE'}),'StatusSelected','yes','TimeSelected','yes','DeltaTimeSelected','yes','BytePortSelected','no','MessageLengthSelected','no','TriggerPort',struct('Selected','no','TriggerType',0),'UserCoding',struct('Selected','no','InterfaceFile','UserDecodingFile','FcnName','UserDecodeFcn','InportSelected','no','InportWidth',1,'OutportSelected','no','OutportWidth',1),'EnablePortSelected','no','UseRXService','no','BoardType','DS1','BoardNo',2,'ControllerNo',1),'OFF',[]}},'TLCFileName',{{'rtican_rx_message','OFF',[]}})  RTISFcnParameters=struct('SFcnRTICANMessage','struct','TLCFileName','char')  RTIBlockParaDefault=struct('BoardTypeNo',4302,'BoardNo',1,'ChannelNo',1,'Parameters',struct('DataFileSupport',struct('DataFileSelectedMaster',0,'DataFileSelectedLocal',0,'DataFileName','','DataFileDate','','SelectedFile',['<no file selected>']),'Options',struct('StatusSelected',1,'TimeSelected',1,'DeltaTimeSelected',1,'BytePortSelected',0,'MessageLengthSelected',0,'TriggerPort',struct('Selected',0,'TriggerType','rising'),'UserCoding',struct('Selected',0,'InterfaceFile','UserDecodingFile','FcnName','UserDecodeFcn','InportSelected',0,'InportWidth',1,'OutportSelected',0,'OutportWidth',1),'EnablePortSelected',0,'SignalOnPortnameSelected',1,'UseRXService',0),'Message',struct('MsgOnBlocknameSelected',0,'MsgName',['RX Message'],'MsgIdFormat',0,'MsgId',100,'MsgLength',8,'NumSignals',1,'SampleTime',-1,'Signal',struct('SgnName',['RX signal'],'SgnStartBit',0,'SgnLength',8,'SgnType',0,'ModeValue',-1,'DataType',0,'SLDataType','SS_DOUBLE','ByteLayout',0,'Factor',1,'Offset',0,'Min',0,'Max',255,'SgnComment',{{}},'SgnUnit',''),'MsgIdNumFormat',0,'MsgComment',{{''}}),'Version',1.2,'general',struct('isFromLib',1)),'GroupId',struct('Group',{{'RTICAN'}},'No',1,'Behavior',{{'NAMECHANGE'}},'BlockType',{{'SINK'}},'NameChangeFlag',0),'SFcnRTICANMessage',struct('MsgType','RX','MsgName',['RX Message'],'MsgIdFormat','STD','MsgId',100,'MsgLength',8,'NumSignals',1,'SampleTime',-1,'Signal',struct('SgnName',['RX signal'],'SgnStartBit',0,'SgnLength',8,'SgnType','standard','ModeValue',-1,'DataType',['unsigned int'],'ByteLayout',['little endian'],'SLDataType','SS_DOUBLE','Factor',1,'Offset',0),'StatusSelected','yes','TimeSelected','yes','DeltaTimeSelected','yes','BytePortSelected','no','MessageLengthSelected','no','EnablePortSelected','no','UserCoding',struct('Selected','no','InterfaceFile','UserDecodingFile','FcnName','UserDecodeFcn','InportSelected','no','InportWidth',1,'OutportSelected','no','OutportWidth',1),'TriggerPort',struct('Selected','no','TriggerType','rising'),'UseRXService','no','BoardType','DS4302','BoardNo',1,'ControllerNo',1,'SFcnPortType','Scalar'),'TLCFileName','rtican_rx_message')
      settings: AttributesFormatString=Group Id: RTICAN2\n  SourceProductName=dSPACE RTI CAN Blockset
  Terminator{,1..5} (6 alike) : Terminator
  Out1 : Outport
  wires:
  FRS_Obj_18_Part1of2/15 -> Terminator2/1
  FRS_Obj_18_Part1of2/14 -> Terminator1/1
  FRS_Obj_18_Part1of2/13 -> Terminator/1
  FRS_Obj_18_Part2of2/10 -> Terminator4/1
  FRS_Obj_18_Part2of2/9 -> Terminator3/1
  FRS_Obj_18_Part2of2/11 -> Terminator5/1
  Bus Creator1/1 -> Out1/1
  FRS_Obj_18_Part1of2/1 -> Bus Creator1/1  "FRS_P1_18_Msg_CheckSum"
  FRS_Obj_18_Part1of2/2 -> Bus Creator1/2  "FRS_P1_18_Msg_AliveCounter"
  FRS_Obj_18_Part1of2/3 -> Bus Creator1/3  "FRS_P1_18_Obj_ExstProb"
  FRS_Obj_18_Part1of2/4 -> Bus Creator1/4  "FRS_P1_18_Obj_XVelRel_Stdev"
  FRS_Obj_18_Part1of2/5 -> Bus Creator1/5  "FRS_P1_18_Obj_XAccRel"
  FRS_Obj_18_Part1of2/6 -> Bus Creator1/6  "FRS_P1_18_Obj_ObstacleProb"
  FRS_Obj_18_Part1of2/7 -> Bus Creator1/7  "FRS_P1_18_Obj_MotionPattern"
  FRS_Obj_18_Part1of2/8 -> Bus Creator1/8  "FRS_P1_18_Obj_YPos_Stdev"
  FRS_Obj_18_Part1of2/9 -> Bus Creator1/9  "FRS_P1_18_Obj_ValidFlag"
  FRS_Obj_18_Part1of2/10 -> Bus Creator1/10  "FRS_P1_18_Obj_XPos_Stdev"
  FRS_Obj_18_Part1of2/11 -> Bus Creator1/11  "FRS_P1_18_Obj_UpdateFlag"
  FRS_Obj_18_Part1of2/12 -> Bus Creator1/12  "FRS_P1_18_Obj_ID"
  FRS_Obj_18_Part2of2/8 -> Bus Creator1/20  "FRS_P2_18_Obj_XVelRel"
  FRS_Obj_18_Part2of2/7 -> Bus Creator1/19  "FRS_P2_18_Obj_YPos"
  FRS_Obj_18_Part2of2/6 -> Bus Creator1/18  "FRS_P2_18_Obj_XPos"
  FRS_Obj_18_Part2of2/5 -> Bus Creator1/17  "FRS_P2_18_Obj_Type"
  FRS_Obj_18_Part2of2/4 -> Bus Creator1/16  "FRS_P2_18_Obj_YVelRel"
  FRS_Obj_18_Part2of2/3 -> Bus Creator1/15  "FRS_P2_18_Obj_MeasFlag"
  FRS_Obj_18_Part2of2/2 -> Bus Creator1/14  "FRS_P2_18_Msg_AliveCounter"
  FRS_Obj_18_Part2of2/1 -> Bus Creator1/13  "FRS_P2_18_Msg_CheckSum"
